simulink model "DC_lead_compensator"  (R2021a)
settings: Solver=VariableStepAuto  StartTime=0.0  StopTime=0.5  MaxStep=1e-4  RelTol=1e-3
values from neighbouring files (symbols this model uses):
  gr = 1024    [DC_twin_parameters.m]
  J = 2.56e4    (= 25600)    [Apollo_LM_design_discrete_observer.m]    (also in Apollo_LM_design_observer.m; Apollo_LM_observer_feedback.m; Apollo_LM_state_feedback.m; DC_twin_parameters.m = 22.8675707733)
  K = K_a    [Apollo_LM_design_observer.m]    (also in Apollo_LM_observer_feedback.m = [k1;k2;k3])
  k = Vnom / w_no_load    (= 0.0309706916287)    [DC_twin_parameters.m]    (also in partial_exam_facit.m = 2)
  k1 = n^3/tauc^3/gM    (= 617.283950617)    [Apollo_LM_observer_feedback.m]
  L = place(A, B, pd)    [Apollo_LM_design_discrete_observer.m]    (also in Apollo_LM_design_observer.m = L_a; Apollo_LM_observer_feedback.m = [l1, l2, l3]; Apollo_LM_state_feedback.m = [l1, l2, l3]; DC_twin_parameters.m = 0.000268)
  R = 1.75    [DC_twin_parameters.m]
undefined symbols (not defined in the file or in its folder): alphad, b, taudc, Td
settings Model: Creator=kjartan  LastModifiedBy=kjartan

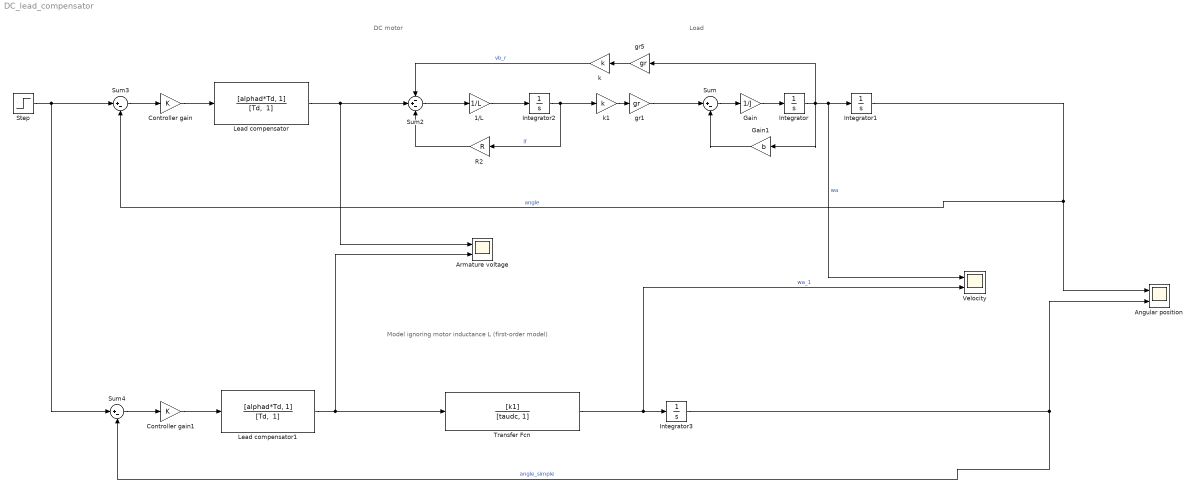
== system DC_lead_compensator ==
  note: Model ignoring motor inductance L (first-order model)
  note: Load
  note: DC motor
  1/L : Gain  Gain=1/L
  Angular position : Scope  NumInputPorts=2
  Armature voltage : Scope  NumInputPorts=2
  Controller gain : Gain  Gain=K
  Controller gain1 : Gain  Gain=K
  Gain : Gain  Gain=1/J
  Gain1 : Gain  Gain=b
  Integrator{,1..3} (4 alike) : Integrator
  Lead compensator : TransferFcn  Numerator=[alphad*Td, 1]  Denominator="[Td,  1]"
  Lead compensator1 : TransferFcn  Numerator=[alphad*Td, 1]  Denominator="[Td,  1]"
  R2 : Gain  Gain=R
  Step : Step  Time=0  After=pi/6  SampleTime=0
  Sum : Sum  Inputs=|+-
  Sum2 : Sum  Inputs=-+-
  Sum3 : Sum  Inputs=|+-
  Sum4 : Sum  Inputs=|+-
  Transfer Fcn : TransferFcn  Numerator=[k1]  Denominator=[taudc, 1]
  Velocity : Scope  NumInputPorts=2
  gr1 : Gain  Gain=gr
  gr5 : Gain  Gain=gr
  k : Gain  Gain=k
  k1 : Gain  Gain=k
  wires:
  gr5/1 -> k/1
  R2/1 -> Sum2/3
  Integrator2/1 -> R2/1, k1/1  "if"
  Sum2/1 -> 1/L/1
  k1/1 -> gr1/1
  1/L/1 -> Integrator2/1
  k/1 -> Sum2/1  "vb_r"
  gr1/1 -> Sum/1
  Gain/1 -> Integrator/1
  Integrator/1 -> Gain1/1, gr5/1, Velocity/1, Integrator1/1  "wa"
  Integrator1/1 -> Angular position/1, Sum3/2  "angle"
  Transfer Fcn/1 -> Velocity/2, Integrator3/1  "wa_1"
  Integrator3/1 -> Angular position/2, Sum4/2  "angle_simple"
  Controller gain/1 -> Lead compensator/1
  Sum3/1 -> Controller gain/1
  Step/1 -> Sum4/1, Sum3/1
  Controller gain1/1 -> Lead compensator1/1
  Sum4/1 -> Controller gain1/1
  Lead compensator1/1 -> Transfer Fcn/1, Armature voltage/2
  Lead compensator/1 -> Sum2/2, Armature voltage/1
  Sum/1 -> Gain/1
  Gain1/1 -> Sum/2
